simulink model "Modelo2"  (R2022a)
settings: configuration reference "MainConfig" (kept outside this file)
PostLoadFcn:
  | load('input_modelo_bateria.mat')
undefined symbols (not defined in the file or in its folder): rest_time, SOC_MAX, SOC_MIN, Temperature
settings Model: PacingRate=1000  Creator=eduardo.guimaraes  LastModifiedBy=mateu
settings ConfigSetRef: SourceName=MainConfig  SourceLocation=Base Workspace

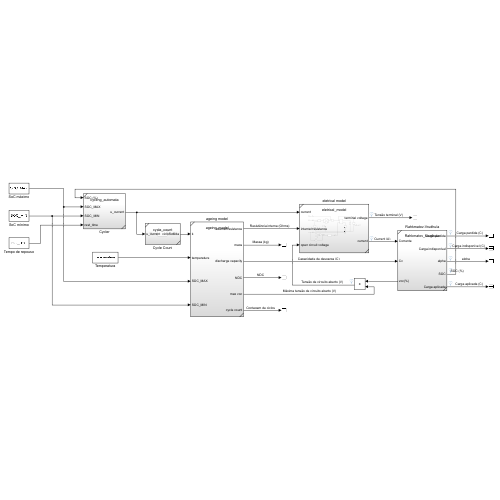
[thumbnail: Simulink's stored preview of the top-level diagram]
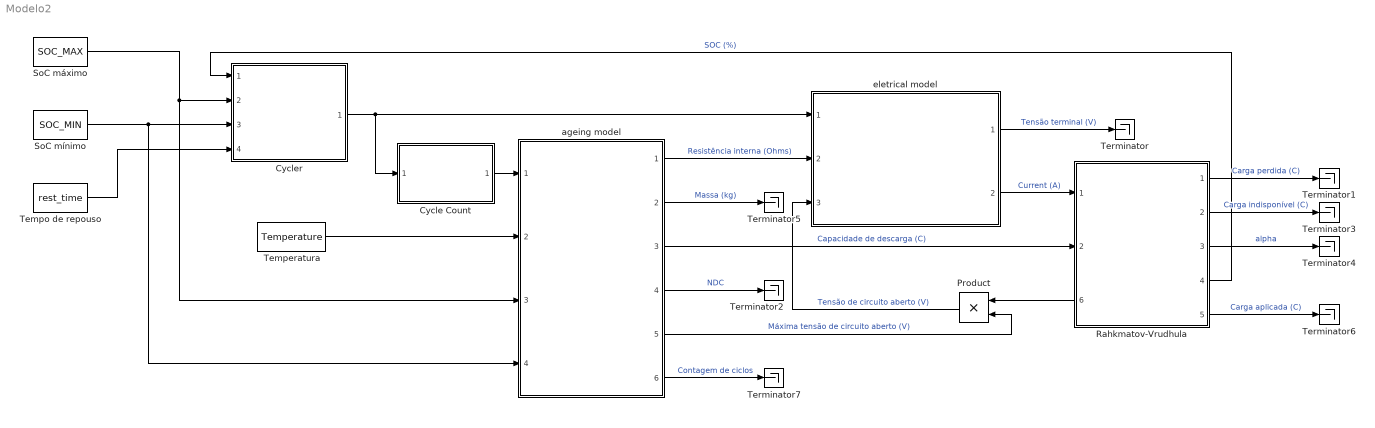
== system Modelo2 ==
  Cycle Count : Subsystem  ReferencedSubsystem=cycle_count
  Cycler : Subsystem  ReferencedSubsystem=cycling_automata
  Product : Product
  Rahkmatov-Vrudhula : Subsystem  ReferencedSubsystem=Rahkmatov_Vrudhula
      settings: PortSchema="{\"entries\":[{\"content\":{\"sides\":[{\"content\":{\"connectorIds\":[\"In1\",\"In2\",\"Out6\"]},\"type\":\"ConnectorPlacement.EquallySpacedRectSide\",\"uuid\":\"83f3e873-db9f-47d1-b7c3-7eda48a10b32\"},{\"content\":{\"connectorIds\":[\"Out1\",\"Out2\",\"Out3\",\"Out4\",\"Out5\"],\"side\":\"RIGHT\"},\"type\":\"ConnectorPlacement.EquallySpacedRectSide\",\"uuid\":\"48ac6012-cdb4-4752-bc48-afa50bea9f0a\"},{\"content\":{\"connectorIds\":[],\"side\":\"TOP\"},\"type\":\"ConnectorPlacement.EquallySpacedRectSide\",\"uuid\":\"9cdc78bf-a718-48f1-92e6-e4070151caee\"}]},\"type\":\"ConnectorPlacement.EquallySpacedConnector\",\"uuid\":\"a231f58d-8e16-4cb4-bc80-61541bcf90eb\"}],\"packageUris\":[\"http://schema.mathworks.com/mf0/Connector/R2020b\"],\"version\":\"1.0\"}"
  SoC máximo : Constant  Value=SOC_MAX
  SoC mínimo : Constant  Value=SOC_MIN
  Temperatura : Constant  Value=Temperature
  Tempo de repouso : Constant  Value=rest_time
  Terminator{,1..7} (8 alike) : Terminator
  ageing model : Subsystem  ReferencedSubsystem=ageing_model
  eletrical model : Subsystem  ReferencedSubsystem=eletrical_model
  wires:
  Temperatura/1 -> ageing model/2
  ageing model/3 -> Rahkmatov-Vrudhula/2  "Capacidade de descarga (C)"
  SoC máximo/1 -> ageing model/3, Cycler/2
  SoC mínimo/1 -> ageing model/4, Cycler/3
  eletrical model/2 -> Rahkmatov-Vrudhula/1  "Current (A)"
  ageing model/1 -> eletrical model/2  "Resistência interna (Ohms)"
  Rahkmatov-Vrudhula/6 -> Product/1
  ageing model/5 -> Product/2  "Máxima tensão de circuito aberto (V)"
  Product/1 -> eletrical model/3  "Tensão de circuito aberto (V)"
  eletrical model/1 -> Terminator/1  "Tensão terminal (V)"
  Rahkmatov-Vrudhula/1 -> Terminator1/1  "Carga perdida (C)"
  Rahkmatov-Vrudhula/2 -> Terminator3/1  "Carga indisponível (C)"
  Rahkmatov-Vrudhula/3 -> Terminator4/1  "alpha"
  ageing model/4 -> Terminator2/1  "NDC"
  ageing model/2 -> Terminator5/1  "Massa (kg)"
  Rahkmatov-Vrudhula/5 -> Terminator6/1  "Carga aplicada (C)"
  ageing model/6 -> Terminator7/1  "Contagem de ciclos"
  Cycler/1 -> eletrical model/1, Cycle Count/1
  Tempo de repouso/1 -> Cycler/4
  Rahkmatov-Vrudhula/4 -> Cycler/1  "SOC (%)"
  Cycle Count/1 -> ageing model/1
